simulink model "myDrive"  (R2021a)
settings: Solver=FixedStepAuto  StartTime=0.0  StopTime=inf  RelTol=1e-3  EnableMultiTasking=on
PreLoadFcn:
  | Ts = 0.01;
  | Ts_wifi = 0.1;
libraries: arduinomotorcarrierlib x3
settings Model: SimulationMode=external  ExtModeTrigDuration=2  Creator=bnewman  LastModifiedBy=danie
settings SolverCC: AlgebraicLoopSolver=TrustRegion
settings DataIOCC: ReturnWorkspaceOutputs=off
settings OptimizationCC: PassReuseOutputArgsThreshold=0  MaxStackSize=64
settings DebuggingCC: ParameterTunabilityLossMsg=error  SFMachineParentedDataDiag=warning  ArithmeticOperatorsInVariantConditions=warning
settings HardwareCC: ProdBitPerPointer=32  ProdBitPerSizeT=32  ProdBitPerPtrDiffT=32  ProdLargestAtomicInteger=Long  ProdLargestAtomicFloat=Double  ProdWordSize=32  ProdHWDeviceType=ARM Compatible->ARM Cortex  UseEmbeddedCoderFeatures=off  UseSimulinkCoderFeatures=off
settings SFSimCC: SimUseLocalCustomCode=off  MATLABDynamicMemAlloc=off  CustomCodeUndefinedFunction=UseInterfaceOnly
settings RTWCC: SystemTargetFile=ert.tlc  HardwareBoard=Arduino MKR1000  TemplateMakefile=ert_default_tmf  GenerateReport=on  RTWUseLocalCustomCode=off  Toolchain=Arduino ARM  BuildConfiguration=Faster Runs  LaunchReport=on
settings CodeAppCC: ForceParamTrailComments=on  OperatorAnnotations=on
settings ERTTargetCC: ERTCustomFileBanners=off  SupportContinuousTime=on  SupportNonInlinedSFcns=on  RemoveResetFunc=off  SupportVariableSizeSignals=on  ModelStepFunctionPrototypeControlCompliant=off

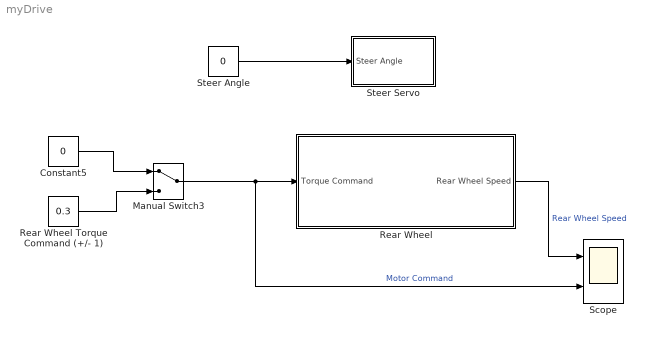
== system myDrive ==
  Constant5 : Constant  Value=0
  Manual Switch3 : ManualSwitch
  Rear Wheel : Subsystem
  Rear Wheel Torque Command (+/- 1) : Constant  Value=0.3
  Scope : Scope  NumInputPorts=2
  Steer Angle : Constant  Value=0
  Steer Servo : Subsystem
  wires:
  Manual Switch3/1 -> Rear Wheel/1(Torque Command), Scope/2  "Motor Command"
  Constant5/1 -> Manual Switch3/1
  Rear Wheel Torque Command (+/- 1)/1 -> Manual Switch3/2
  Rear Wheel/1(Rear Wheel Speed) -> Scope/1  "Rear Wheel Speed"
  Steer Angle/1 -> Steer Servo/1(Steer Angle)

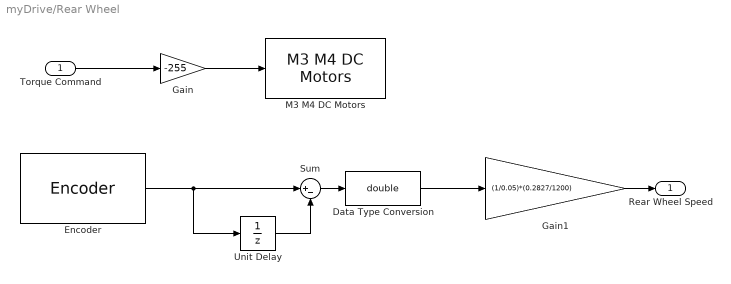
== system myDrive/Rear Wheel ==
  Torque Command : Inport
  Data Type Conversion : DataTypeConversion  OutDataTypeStr=double
  Encoder : arduinomotorcarrierlib/Encoder  SlaveAddress=uint8( hex2dec( '66' ) )  blockPlatform=ARDUINO  Encoder=2  ShowSpeed=off  ResetOption=on  SampleTime=0.05
      settings: SourceProductBaseCode=ARDUINO
  Gain : Gain  Gain=-255
  Gain1 : Gain  Gain=(1/0.05)*(0.2827/1200)
  M3 M4 DC Motors : arduinomotorcarrierlib/M3 M4 DC Motors  MotorNumber=M4  forwardPinNumber=4  reversePinNumber=5
      settings: SourceProductBaseCode=ARDUINO
  Sum : Sum  Inputs=|+-
  Unit Delay : UnitDelay  SampleTime=-1  HasFrameUpgradeWarning=on
  Rear Wheel Speed : Outport
  wires:
  Gain/1 -> M3 M4 DC Motors/1
  Torque Command/1 -> Gain/1
  Sum/1 -> Data Type Conversion/1
  Unit Delay/1 -> Sum/2
  Data Type Conversion/1 -> Gain1/1
  Encoder/1 -> Sum/1, Unit Delay/1
  Gain1/1 -> Rear Wheel Speed/1

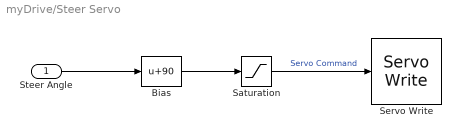
== system myDrive/Steer Servo ==
  Steer Angle : Inport
  Bias : Bias  Bias=90
  Saturation : Saturate  UpperLimit=120  LowerLimit=60
  Servo Write : arduinomotorcarrierlib/Servo Write  SlaveAddress=uint8( hex2dec( '66' ) )  blockPlatform=ARDUINO  MotorNumber=3  MotorCarrierPWMFreq=100
      settings: SourceProductBaseCode=ARDUINO
  wires:
  Bias/1 -> Saturation/1
  Saturation/1 -> Servo Write/1  "Servo Command"
  Steer Angle/1 -> Bias/1
